simulink model "kurtosis"  (R2012b)
settings: Solver=ode45  StartTime=0.0  StopTime=3171  RelTol=1e-3
libraries: xbsIndex_r4 x3174, casper_library_flow_control x64, casper_library_misc x1, simulink_xsg_bridge x1
(part 7 of 24)

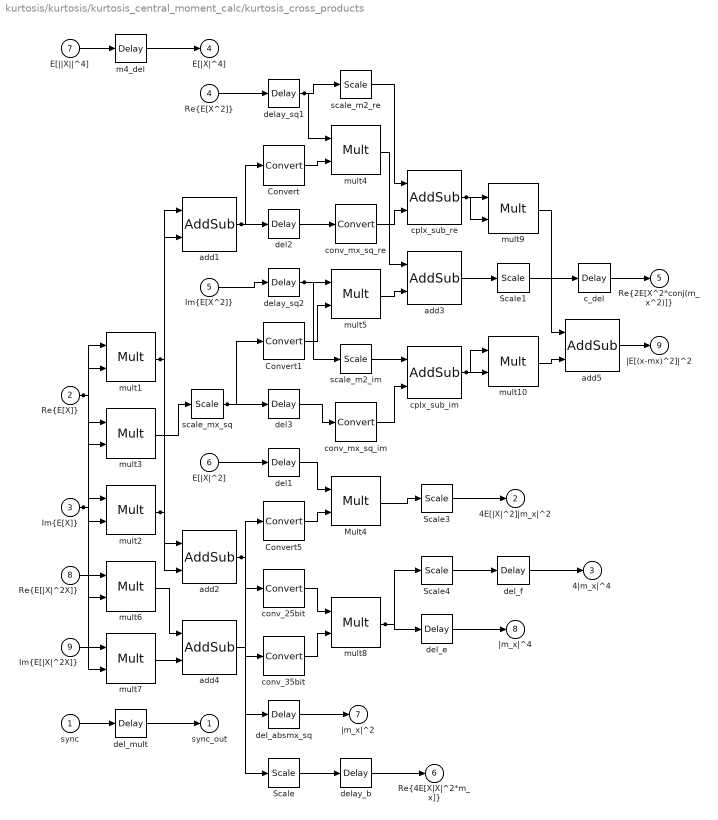
== system kurtosis/kurtosis/kurtosis_central_moment_calc/kurtosis_cross_products ==
  sync : Inport
  "Re{E[X]}" : Inport  Port=2
  "Im{E[X]}" : Inport  Port=3
  "Re{E[X^2]}" : Inport  Port=4
  "Im{E[X^2]}" : Inport  Port=5
  E[|X|^2] : Inport  Port=6
  E[||X||^4] : Inport  Port=7
  "Re{E[|X|^2X]}" : Inport  Port=8
  "Im{E[|X|^2X]}" : Inport  Port=9
  Convert : xbsIndex_r4/Convert  gui_display_data_type=Fixed-point  arith_type="Signed  (2's comp)"  n_bits=25  bin_pt=22  float_type=Single  exp_bits=8  fraction_bits=24  quantization="Round  (unbiased: +/- Inf)"  overflow=Saturate  en=off  latency=1  dbl_ovrd=off  pipeline=off  block_type=convert
  Convert1 : xbsIndex_r4/Convert  gui_display_data_type=Fixed-point  arith_type="Signed  (2's comp)"  n_bits=25  bin_pt=22  float_type=Single  exp_bits=8  fraction_bits=24  quantization="Round  (unbiased: +/- Inf)"  overflow=Saturate  en=off  latency=1  dbl_ovrd=off  pipeline=off  block_type=convert
  Convert5 : xbsIndex_r4/Convert  gui_display_data_type=Fixed-point  arith_type="Signed  (2's comp)"  n_bits=25  bin_pt=22  float_type=Single  exp_bits=8  fraction_bits=24  quantization="Round  (unbiased: +/- Inf)"  overflow=Saturate  en=off  latency=5  dbl_ovrd=off  pipeline=off  block_type=convert
  Mult4 : xbsIndex_r4/Mult  precision=Full  arith_type="Signed  (2's comp)"  n_bits=36  bin_pt=34  quantization=Truncate  overflow=Wrap  en=off  latency=5  dbl_ovrd=off  use_behavioral_HDL=off  opt=Speed  use_embedded=on  optimum_pipeline=off  pipeline=on  use_rpm=on  placement_style=Triangular  block_type=mult
  Scale : xbsIndex_r4/Scale  scale_factor=2  dbl_ovrd=off  block_type=scale
  Scale1 : xbsIndex_r4/Scale  scale_factor=1  dbl_ovrd=off  block_type=scale
  Scale3 : xbsIndex_r4/Scale  scale_factor=2  dbl_ovrd=off  block_type=scale
  Scale4 : xbsIndex_r4/Scale  scale_factor=2  dbl_ovrd=off  block_type=scale
  add1 : xbsIndex_r4/AddSub  mode=Subtraction  use_carryin=off  use_carryout=off  en=off  latency=2  precision=Full  arith_type="Signed  (2's comp)"  n_bits=36  bin_pt=34  quantization=Truncate  overflow=Wrap  dbl_ovrd=off  use_behavioral_HDL=off  hw_selection=Fabric  pipelined=off  block_type=addsub
  add2 : xbsIndex_r4/AddSub  mode=Addition  use_carryin=off  use_carryout=off  en=off  latency=2  precision=Full  arith_type="Signed  (2's comp)"  n_bits=36  bin_pt=34  quantization=Truncate  overflow=Wrap  dbl_ovrd=off  use_behavioral_HDL=off  hw_selection=Fabric  pipelined=off  block_type=addsub
  add3 : xbsIndex_r4/AddSub  mode=Addition  use_carryin=off  use_carryout=off  en=off  latency=2  precision=Full  arith_type="Signed  (2's comp)"  n_bits=36  bin_pt=34  quantization=Truncate  overflow=Wrap  dbl_ovrd=off  use_behavioral_HDL=off  hw_selection=Fabric  pipelined=off  block_type=addsub
  add4 : xbsIndex_r4/AddSub  mode=Addition  use_carryin=off  use_carryout=off  en=off  latency=2  precision=Full  arith_type="Signed  (2's comp)"  n_bits=36  bin_pt=34  quantization=Truncate  overflow=Wrap  dbl_ovrd=off  use_behavioral_HDL=off  hw_selection=Fabric  pipelined=off  block_type=addsub
  add5 : xbsIndex_r4/AddSub  mode=Addition  use_carryin=off  use_carryout=off  en=off  latency=3  precision=Full  arith_type="Signed  (2's comp)"  n_bits=36  bin_pt=34  quantization=Truncate  overflow=Wrap  dbl_ovrd=off  use_behavioral_HDL=off  hw_selection=Fabric  pipelined=off  block_type=addsub
  c_del : xbsIndex_r4/Delay  rst=off  infoeditControl=Selection of Reset will increase slice count due to use of real FFs and instead of SRLs  en=off  latency=4  dbl_ovrd=off  reg_retiming=off  block_type=delay
  conv_25bit : xbsIndex_r4/Convert  gui_display_data_type=Fixed-point  arith_type="Signed  (2's comp)"  n_bits=25  bin_pt=22  float_type=Single  exp_bits=8  fraction_bits=24  quantization="Round  (unbiased: +/- Inf)"  overflow=Saturate  en=off  latency=3  dbl_ovrd=off  pipeline=off  block_type=convert
  conv_35bit : xbsIndex_r4/Convert  gui_display_data_type=Fixed-point  arith_type="Signed  (2's comp)"  n_bits=35  bin_pt=32  float_type=Single  exp_bits=8  fraction_bits=24  quantization="Round  (unbiased: +/- Inf)"  overflow=Saturate  en=off  latency=3  dbl_ovrd=off  pipeline=off  block_type=convert
  conv_mx_sq_im : xbsIndex_r4/Convert  gui_display_data_type=Fixed-point  arith_type="Signed  (2's comp)"  n_bits=35  bin_pt=32  float_type=Single  exp_bits=8  fraction_bits=24  quantization="Round  (unbiased: +/- Inf)"  overflow=Saturate  en=off  latency=0  dbl_ovrd=off  pipeline=off  block_type=convert
  conv_mx_sq_re : xbsIndex_r4/Convert  gui_display_data_type=Fixed-point  arith_type="Signed  (2's comp)"  n_bits=35  bin_pt=32  float_type=Single  exp_bits=8  fraction_bits=24  quantization="Round  (unbiased: +/- Inf)"  overflow=Saturate  en=off  latency=0  dbl_ovrd=off  pipeline=off  block_type=convert
  cplx_sub_im : xbsIndex_r4/AddSub  mode=Subtraction  use_carryin=off  use_carryout=off  en=off  latency=2  precision=Full  arith_type="Signed  (2's comp)"  n_bits=36  bin_pt=34  quantization=Truncate  overflow=Wrap  dbl_ovrd=off  use_behavioral_HDL=off  hw_selection=Fabric  pipelined=off  block_type=addsub
  cplx_sub_re : xbsIndex_r4/AddSub  mode=Subtraction  use_carryin=off  use_carryout=off  en=off  latency=2  precision=Full  arith_type="Signed  (2's comp)"  n_bits=36  bin_pt=34  quantization=Truncate  overflow=Wrap  dbl_ovrd=off  use_behavioral_HDL=off  hw_selection=Fabric  pipelined=off  block_type=addsub
  del1 : xbsIndex_r4/Delay  rst=off  infoeditControl=Selection of Reset will increase slice count due to use of real FFs and instead of SRLs  en=off  latency=10  dbl_ovrd=off  reg_retiming=off  block_type=delay
  del2 : xbsIndex_r4/Delay  rst=off  infoeditControl=Selection of Reset will increase slice count due to use of real FFs and instead of SRLs  en=off  latency=1  dbl_ovrd=off  reg_retiming=off  block_type=delay
  del3 : xbsIndex_r4/Delay  rst=off  infoeditControl=Selection of Reset will increase slice count due to use of real FFs and instead of SRLs  en=off  latency=1  dbl_ovrd=off  reg_retiming=off  block_type=delay
  del_absmx_sq : xbsIndex_r4/Delay  rst=off  infoeditControl=Selection of Reset will increase slice count due to use of real FFs and instead of SRLs  en=off  latency=10  dbl_ovrd=off  reg_retiming=off  block_type=delay
  del_e : xbsIndex_r4/Delay  rst=off  infoeditControl=Selection of Reset will increase slice count due to use of real FFs and instead of SRLs  en=off  latency=2  dbl_ovrd=off  reg_retiming=off  block_type=delay
  del_f : xbsIndex_r4/Delay  rst=off  infoeditControl=Selection of Reset will increase slice count due to use of real FFs and instead of SRLs  en=off  latency=2  dbl_ovrd=off  reg_retiming=off  block_type=delay
  del_mult : xbsIndex_r4/Delay  rst=off  infoeditControl=Selection of Reset will increase slice count due to use of real FFs and instead of SRLs  en=off  latency=15  dbl_ovrd=off  reg_retiming=off  block_type=delay
  delay_b : xbsIndex_r4/Delay  rst=off  infoeditControl=Selection of Reset will increase slice count due to use of real FFs and instead of SRLs  en=off  latency=7  dbl_ovrd=off  reg_retiming=off  block_type=delay
  delay_sq1 : xbsIndex_r4/Delay  rst=off  infoeditControl=Selection of Reset will increase slice count due to use of real FFs and instead of SRLs  en=off  latency=6  dbl_ovrd=off  reg_retiming=off  block_type=delay
  delay_sq2 : xbsIndex_r4/Delay  rst=off  infoeditControl=Selection of Reset will increase slice count due to use of real FFs and instead of SRLs  en=off  latency=6  dbl_ovrd=off  reg_retiming=off  block_type=delay
  m4_del : xbsIndex_r4/Delay  rst=off  infoeditControl=Selection of Reset will increase slice count due to use of real FFs and instead of SRLs  en=off  latency=15  dbl_ovrd=off  reg_retiming=off  block_type=delay
  mult{1..2,4..5} (4 alike) : xbsIndex_r4/Mult  precision=Full  arith_type="Signed  (2's comp)"  n_bits=36  bin_pt=34  quantization=Truncate  overflow=Wrap  en=off  latency=3  dbl_ovrd=off  use_behavioral_HDL=off  opt=Speed  use_embedded=on  optimum_pipeline=off  pipeline=on  use_rpm=on  placement_style=Triangular  block_type=mult
  mult10 : xbsIndex_r4/Mult  precision=Full  arith_type="Signed  (2's comp)"  n_bits=36  bin_pt=34  quantization=Truncate  overflow=Wrap  en=off  latency=4  dbl_ovrd=off  use_behavioral_HDL=off  opt=Speed  use_embedded=on  optimum_pipeline=off  pipeline=on  use_rpm=on  placement_style=Triangular  block_type=mult
  mult3 : xbsIndex_r4/Mult  precision=Full  arith_type="Signed  (2's comp)"  n_bits=36  bin_pt=34  quantization=Truncate  overflow=Wrap  en=off  latency=5  dbl_ovrd=off  use_behavioral_HDL=off  opt=Speed  use_embedded=on  optimum_pipeline=off  pipeline=on  use_rpm=on  placement_style=Triangular  block_type=mult
  mult6 : xbsIndex_r4/Mult  precision=Full  arith_type="Signed  (2's comp)"  n_bits=36  bin_pt=34  quantization=Truncate  overflow=Wrap  en=off  latency=6  dbl_ovrd=off  use_behavioral_HDL=off  opt=Speed  use_embedded=on  optimum_pipeline=off  pipeline=on  use_rpm=on  placement_style=Triangular  block_type=mult
  mult7 : xbsIndex_r4/Mult  precision=Full  arith_type="Signed  (2's comp)"  n_bits=36  bin_pt=34  quantization=Truncate  overflow=Wrap  en=off  latency=6  dbl_ovrd=off  use_behavioral_HDL=off  opt=Speed  use_embedded=on  optimum_pipeline=off  pipeline=on  use_rpm=on  placement_style=Triangular  block_type=mult
  mult8 : xbsIndex_r4/Mult  precision=Full  arith_type="Signed  (2's comp)"  n_bits=36  bin_pt=34  quantization=Truncate  overflow=Wrap  en=off  latency=5  dbl_ovrd=off  use_behavioral_HDL=off  opt=Speed  use_embedded=on  optimum_pipeline=off  pipeline=on  use_rpm=on  placement_style=Triangular  block_type=mult
  mult9 : xbsIndex_r4/Mult  precision=Full  arith_type="Signed  (2's comp)"  n_bits=36  bin_pt=34  quantization=Truncate  overflow=Wrap  en=off  latency=4  dbl_ovrd=off  use_behavioral_HDL=off  opt=Speed  use_embedded=on  optimum_pipeline=off  pipeline=on  use_rpm=on  placement_style=Triangular  block_type=mult
  scale_m2_im : xbsIndex_r4/Scale  scale_factor=-10  dbl_ovrd=off  block_type=scale
  scale_m2_re : xbsIndex_r4/Scale  scale_factor=-10  dbl_ovrd=off  block_type=scale
  scale_mx_sq : xbsIndex_r4/Scale  scale_factor=1  dbl_ovrd=off  block_type=scale
  sync_out : Outport
  4E[|X|^2]|m_x|^2 : Outport  Port=2
  4|m_x|^4 : Outport  Port=3
  E[|X|^4] : Outport  Port=4
  "Re{2E[X^2*conj(m_x^2)]}" : Outport  Port=5
  "Re{4E[X|X|^2*m_x]}" : Outport  Port=6
  |m_x|^2 : Outport  Port=7
  |m_x|^4 : Outport  Port=8
  |E[(x-mx)^2]|^2 : Outport  Port=9
  wires:
  "Re{E[X]}"/1 -> mult6/2, mult3/1, mult1/2, mult1/1
  "Im{E[X]}"/1 -> mult7/2, mult3/2, mult2/2, mult2/1
  mult1/1 -> add2/1, add1/1
  mult2/1 -> add2/2, add1/2
  add1/1 -> del2/1, Convert/1
  scale_mx_sq/1 -> del3/1, Convert1/1
  delay_sq1/1 -> scale_m2_re/1, mult4/1
  delay_sq2/1 -> scale_m2_im/1, mult5/1
  add2/1 -> del_absmx_sq/1, Convert5/1, conv_35bit/1, conv_25bit/1
  mult8/1 -> Scale4/1, del_e/1
  cplx_sub_re/1 -> mult9/2, mult9/1
  cplx_sub_im/1 -> mult10/2, mult10/1
  del_absmx_sq/1 -> |m_x|^2/1
  add5/1 -> |E[(x-mx)^2]|^2/1
  del_f/1 -> 4|m_x|^4/1
  del_e/1 -> |m_x|^4/1
  Scale3/1 -> 4E[|X|^2]|m_x|^2/1
  c_del/1 -> "Re{2E[X^2*conj(m_x^2)]}"/1
  delay_b/1 -> "Re{4E[X|X|^2*m_x]}"/1
  m4_del/1 -> E[|X|^4]/1
  E[||X||^4]/1 -> m4_del/1
  del_mult/1 -> sync_out/1
  sync/1 -> del_mult/1
  mult10/1 -> add5/2
  mult9/1 -> add5/1
  conv_mx_sq_im/1 -> cplx_sub_im/2
  scale_m2_im/1 -> cplx_sub_im/1
  conv_mx_sq_re/1 -> cplx_sub_re/2
  scale_m2_re/1 -> cplx_sub_re/1
  del3/1 -> conv_mx_sq_im/1
  del2/1 -> conv_mx_sq_re/1
  Scale4/1 -> del_f/1
  Mult4/1 -> Scale3/1
  Convert5/1 -> Mult4/2
  del1/1 -> Mult4/1
  E[|X|^2]/1 -> del1/1
  Scale1/1 -> c_del/1
  add3/1 -> Scale1/1
  Scale/1 -> delay_b/1
  add4/1 -> Scale/1
  conv_35bit/1 -> mult8/2
  conv_25bit/1 -> mult8/1
  mult7/1 -> add4/2
  mult6/1 -> add4/1
  "Im{E[|X|^2X]}"/1 -> mult7/1
  "Re{E[|X|^2X]}"/1 -> mult6/1
  mult5/1 -> add3/2
  mult4/1 -> add3/1
  Convert1/1 -> mult5/2
  Convert/1 -> mult4/2
  "Im{E[X^2]}"/1 -> delay_sq2/1
  "Re{E[X^2]}"/1 -> delay_sq1/1
  mult3/1 -> scale_mx_sq/1

== system kurtosis/kurtosis/kurtosis_central_moment_calc/kurtosis_den ==
  E[|X|^2] : Inport
  |m_x|^2 : Inport  Port=2
  Sub : xbsIndex_r4/AddSub  mode=Subtraction  use_carryin=off  use_carryout=off  en=off  latency=4  precision=Full  arith_type="Signed  (2's comp)"  n_bits=36  bin_pt=34  quantization=Truncate  overflow=Wrap  dbl_ovrd=off  use_behavioral_HDL=off  hw_selection=Fabric  pipelined=off  block_type=addsub
  conv : xbsIndex_r4/Convert  gui_display_data_type=Fixed-point  arith_type="Signed  (2's comp)"  n_bits=64  bin_pt=56  float_type=Single  exp_bits=8  fraction_bits=24  quantization="Round  (unbiased: +/- Inf)"  overflow=Saturate  en=off  latency=1  dbl_ovrd=off  pipeline=off  block_type=convert
  scale : xbsIndex_r4/Scale  scale_factor=-10  dbl_ovrd=off  block_type=scale
  square : xbsIndex_r4/Mult  precision=Full  arith_type="Signed  (2's comp)"  n_bits=36  bin_pt=34  quantization=Truncate  overflow=Wrap  en=off  latency=5  dbl_ovrd=off  use_behavioral_HDL=off  opt=Speed  use_embedded=on  optimum_pipeline=off  pipeline=on  use_rpm=on  placement_style=Triangular  block_type=mult
  square_conv_25bit : xbsIndex_r4/Convert  gui_display_data_type=Fixed-point  arith_type="Signed  (2's comp)"  n_bits=25  bin_pt=21  float_type=Single  exp_bits=8  fraction_bits=24  quantization="Round  (unbiased: +/- Inf)"  overflow=Saturate  en=off  latency=3  dbl_ovrd=off  pipeline=off  block_type=convert
  square_conv_35bit : xbsIndex_r4/Convert  gui_display_data_type=Fixed-point  arith_type="Signed  (2's comp)"  n_bits=35  bin_pt=31  float_type=Single  exp_bits=8  fraction_bits=24  quantization="Round  (unbiased: +/- Inf)"  overflow=Saturate  en=off  latency=3  dbl_ovrd=off  pipeline=off  block_type=convert
  E[|X-m_x|^2]^2 : Outport
  wires:
  Sub/1 -> square_conv_25bit/1, square_conv_35bit/1
  conv/1 -> E[|X-m_x|^2]^2/1
  square/1 -> conv/1
  square_conv_25bit/1 -> square/2
  square_conv_35bit/1 -> square/1
  |m_x|^2/1 -> Sub/2
  scale/1 -> Sub/1
  E[|X|^2]/1 -> scale/1

== system kurtosis/kurtosis/kurtosis_central_moment_calc/kurtosis_num ==
  sync : Inport
  4E[|X|^2]|m_x|^2 : Inport  Port=2
  4|m_x|^4 : Inport  Port=3
  E[|X|^4] : Inport  Port=4
  "Re{2E[X^2*conj(m_x^2)]}" : Inport  Port=5
  "Re{4E[X|X|^2*m_x]}" : Inport  Port=6
  |m_x|^4 : Inport  Port=7
  |E[(x-mx)^2]|^2 : Inport  Port=8
  a_del : xbsIndex_r4/Delay  rst=off  infoeditControl=Selection of Reset will increase slice count due to use of real FFs and instead of SRLs  en=off  latency=4  dbl_ovrd=off  reg_retiming=off  block_type=delay
  add : xbsIndex_r4/AddSub  mode=Addition  use_carryin=off  use_carryout=off  en=off  latency=4  precision=Full  arith_type="Signed  (2's comp)"  n_bits=36  bin_pt=34  quantization=Truncate  overflow=Wrap  dbl_ovrd=off  use_behavioral_HDL=off  hw_selection=Fabric  pipelined=off  block_type=addsub
  add_aef : xbsIndex_r4/AddSub  mode=Addition  use_carryin=off  use_carryout=off  en=off  latency=4  precision=Full  arith_type="Signed  (2's comp)"  n_bits=36  bin_pt=34  quantization=Truncate  overflow=Wrap  dbl_ovrd=off  use_behavioral_HDL=off  hw_selection=Fabric  pipelined=off  block_type=addsub
  add_dcb : xbsIndex_r4/AddSub  mode=Addition  use_carryin=off  use_carryout=off  en=off  latency=4  precision=Full  arith_type="Signed  (2's comp)"  n_bits=36  bin_pt=34  quantization=Truncate  overflow=Wrap  dbl_ovrd=off  use_behavioral_HDL=off  hw_selection=Fabric  pipelined=off  block_type=addsub
  conv : xbsIndex_r4/Convert  gui_display_data_type=Fixed-point  arith_type="Signed  (2's comp)"  n_bits=96  bin_pt=84  float_type=Single  exp_bits=8  fraction_bits=24  quantization="Round  (unbiased: +/- Inf)"  overflow=Saturate  en=off  latency=1  dbl_ovrd=off  pipeline=off  block_type=convert
  scale_a : xbsIndex_r4/Scale  scale_factor=-10  dbl_ovrd=off  block_type=scale
  scale_b : xbsIndex_r4/Scale  scale_factor=-10  dbl_ovrd=off  block_type=scale
  scale_c : xbsIndex_r4/Scale  scale_factor=-10  dbl_ovrd=off  block_type=scale
  scale_d : xbsIndex_r4/Scale  scale_factor=-10  dbl_ovrd=off  block_type=scale
  sub_cb : xbsIndex_r4/AddSub  mode=Subtraction  use_carryin=off  use_carryout=off  en=off  latency=4  precision=Full  arith_type="Signed  (2's comp)"  n_bits=36  bin_pt=34  quantization=Truncate  overflow=Wrap  dbl_ovrd=off  use_behavioral_HDL=off  hw_selection=Fabric  pipelined=off  block_type=addsub
  sub_dh : xbsIndex_r4/AddSub  mode=Subtraction  use_carryin=off  use_carryout=off  en=off  latency=4  precision=Full  arith_type="Signed  (2's comp)"  n_bits=36  bin_pt=34  quantization=Truncate  overflow=Wrap  dbl_ovrd=off  use_behavioral_HDL=off  hw_selection=Fabric  pipelined=off  block_type=addsub
  sub_ef : xbsIndex_r4/AddSub  mode=Subtraction  use_carryin=off  use_carryout=off  en=off  latency=4  precision=Full  arith_type="Signed  (2's comp)"  n_bits=36  bin_pt=34  quantization=Truncate  overflow=Wrap  dbl_ovrd=off  use_behavioral_HDL=off  hw_selection=Fabric  pipelined=off  block_type=addsub
  sync_del : xbsIndex_r4/Delay  rst=off  infoeditControl=Selection of Reset will increase slice count due to use of real FFs and instead of SRLs  en=off  latency=13  dbl_ovrd=off  reg_retiming=off  block_type=delay
  sync_out : Outport
  E[|X-m_x|^4] : Outport  Port=2
  wires:
  sync_del/1 -> sync_out/1
  conv/1 -> E[|X-m_x|^4]/1
  add/1 -> conv/1
  add_dcb/1 -> add/2
  add_aef/1 -> add/1
  sub_cb/1 -> add_dcb/2
  sub_dh/1 -> add_dcb/1
  a_del/1 -> add_aef/2
  sub_ef/1 -> add_aef/1
  scale_a/1 -> a_del/1
  |E[(x-mx)^2]|^2/1 -> sub_dh/2
  scale_d/1 -> sub_dh/1
  scale_b/1 -> sub_cb/2
  scale_c/1 -> sub_cb/1
  4|m_x|^4/1 -> sub_ef/2
  |m_x|^4/1 -> sub_ef/1
  4E[|X|^2]|m_x|^2/1 -> scale_d/1
  "Re{2E[X^2*conj(m_x^2)]}"/1 -> scale_c/1
  "Re{4E[X|X|^2*m_x]}"/1 -> scale_b/1
  E[|X|^4]/1 -> scale_a/1
  sync/1 -> sync_del/1

== system kurtosis/kurtosis/kurtosis_origin_moments_1/abs_x_sq ==
  c : Inport
  c_to_ri : Subsystem
  imag_square : xbsIndex_r4/Mult  precision=Full  arith_type="Signed  (2's comp)"  n_bits=16  bin_pt=14  quantization=Truncate  overflow=Wrap  en=off  latency=3  dbl_ovrd=off  use_behavioral_HDL=off  opt=Speed  use_embedded=on  optimum_pipeline=off  pipeline=on  use_rpm=on  placement_style=Rectangular shape  block_type=mult
  power_adder : xbsIndex_r4/AddSub  mode=Addition  use_carryin=off  use_carryout=off  en=off  latency=2  precision=Full  arith_type=Unsigned  n_bits=16  bin_pt=14  quantization=Truncate  overflow=Wrap  dbl_ovrd=off  use_behavioral_HDL=on  hw_selection=Fabric  pipelined=off  use_rpm=on  block_type=addsub
  real_square : xbsIndex_r4/Mult  precision=Full  arith_type="Signed  (2's comp)"  n_bits=16  bin_pt=14  quantization=Truncate  overflow=Wrap  en=off  latency=3  dbl_ovrd=off  use_behavioral_HDL=off  opt=Speed  use_embedded=on  optimum_pipeline=off  pipeline=on  use_rpm=on  placement_style=Triangular  block_type=mult
  power : Outport
  wires:
  c_to_ri/2(im) -> imag_square/2, imag_square/1
  c_to_ri/1(re) -> real_square/2, real_square/1
  real_square/1 -> power_adder/1
  power_adder/1 -> power/1
  imag_square/1 -> power_adder/2
  c/1 -> c_to_ri/1(c)

== system kurtosis/kurtosis/kurtosis_origin_moments_1/c_to_ri_xin ==
  c : Inport
  force_im : xbsIndex_r4/Reinterpret  force_arith_type=on  arith_type="Signed  (2's comp)"  force_bin_pt=on  bin_pt=17  block_type=reinterpret
  force_re : xbsIndex_r4/Reinterpret  force_arith_type=on  arith_type="Signed  (2's comp)"  force_bin_pt=on  bin_pt=17  block_type=reinterpret
  slice_im : xbsIndex_r4/Slice  nbits=18  boolean_output=off  mode=Lower Bit Location + Width  bit1=0  base1=MSB of Input  bit0=0  base0=LSB of Input  dbl_ovrd=off  block_type=slice
  slice_re : xbsIndex_r4/Slice  nbits=18  boolean_output=off  mode=Upper Bit Location + Width  bit1=0  base1=MSB of Input  bit0=0  base0=LSB of Input  dbl_ovrd=off  block_type=slice
  re : Outport
  im : Outport  Port=2
  wires:
  c/1 -> slice_im/1, slice_re/1
  force_im/1 -> im/1
  slice_im/1 -> force_im/1
  force_re/1 -> re/1
  slice_re/1 -> force_re/1

== system kurtosis/kurtosis/kurtosis_origin_moments_1/cplx_sq ==
  a : Inport
  b : Inport  Port=2
  AddSub : xbsIndex_r4/AddSub  mode=Subtraction  use_carryin=off  use_carryout=off  en=off  latency=2  precision=Full  arith_type=Unsigned  n_bits=16  bin_pt=14  quantization=Truncate  overflow=Wrap  dbl_ovrd=off  use_behavioral_HDL=on  hw_selection=Fabric  pipelined=off  block_type=addsub
  AddSub1 : xbsIndex_r4/AddSub  mode=Addition  use_carryin=off  use_carryout=off  en=off  latency=2  precision=Full  arith_type=Unsigned  n_bits=16  bin_pt=14  quantization=Truncate  overflow=Wrap  dbl_ovrd=off  use_behavioral_HDL=on  hw_selection=Fabric  pipelined=off  block_type=addsub
  a_input_c_to_ri : Subsystem
  b_input_c_to_ri : Subsystem
  c_output_ri_to_c : Subsystem
  convert0 : xbsIndex_r4/Convert  gui_display_data_type=Fixed-point  arith_type="Signed  (2's comp)"  n_bits=37  bin_pt=34  float_type=Single  exp_bits=8  fraction_bits=24  quantization=Truncate  overflow=Wrap  en=off  latency=1  dbl_ovrd=off  pipeline=on  block_type=convert
  convert1 : xbsIndex_r4/Convert  gui_display_data_type=Fixed-point  arith_type="Signed  (2's comp)"  n_bits=37  bin_pt=34  float_type=Single  exp_bits=8  fraction_bits=24  quantization=Truncate  overflow=Wrap  en=off  latency=1  dbl_ovrd=off  pipeline=on  block_type=convert
  mults : Subsystem
  c : Outport
  wires:
  a_input_c_to_ri/1(re) -> mults/7(a4), mults/1(a1)  "a_re"
  b_input_c_to_ri/1(re) -> mults/6(b3), mults/2(b1)  "b_re"
  a_input_c_to_ri/2(im) -> mults/5(a3), mults/3(a2)  "a_im"
  b_input_c_to_ri/2(im) -> mults/8(b4), mults/4(b2)  "b_im"
  convert1/1 -> c_output_ri_to_c/2(im)  "c_im"
  AddSub1/1 -> convert1/1
  convert0/1 -> c_output_ri_to_c/1(re)  "c_re"
  AddSub/1 -> convert0/1
  mults/4(c4) -> AddSub1/2
  mults/3(c3) -> AddSub1/1
  mults/2(c2) -> AddSub/2
  mults/1(c1) -> AddSub/1
  c_output_ri_to_c/1(c) -> c/1
  b/1 -> b_input_c_to_ri/1(c)
  a/1 -> a_input_c_to_ri/1(c)

== system kurtosis/kurtosis/kurtosis_origin_moments_1/ri_to_c_x_3rd ==
  re : Inport
  im : Inport  Port=2
  concat : xbsIndex_r4/Concat  num_inputs=2  dbl_ovrd=off  block_type=concat
  force_im : xbsIndex_r4/Reinterpret  force_arith_type=on  arith_type=Unsigned  force_bin_pt=on  bin_pt=0  block_type=reinterpret
  force_re : xbsIndex_r4/Reinterpret  force_arith_type=on  arith_type=Unsigned  force_bin_pt=on  bin_pt=0  block_type=reinterpret
  c : Outport
  wires:
  force_re/1 -> concat/1
  re/1 -> force_re/1
  force_im/1 -> concat/2
  im/1 -> force_im/1
  concat/1 -> c/1

== system kurtosis/kurtosis/kurtosis_origin_moments_2/abs_x_sq ==
  c : Inport
  c_to_ri : Subsystem
  imag_square : xbsIndex_r4/Mult  precision=Full  arith_type="Signed  (2's comp)"  n_bits=16  bin_pt=14  quantization=Truncate  overflow=Wrap  en=off  latency=3  dbl_ovrd=off  use_behavioral_HDL=off  opt=Speed  use_embedded=on  optimum_pipeline=off  pipeline=on  use_rpm=on  placement_style=Rectangular shape  block_type=mult
  power_adder : xbsIndex_r4/AddSub  mode=Addition  use_carryin=off  use_carryout=off  en=off  latency=2  precision=Full  arith_type=Unsigned  n_bits=16  bin_pt=14  quantization=Truncate  overflow=Wrap  dbl_ovrd=off  use_behavioral_HDL=on  hw_selection=Fabric  pipelined=off  use_rpm=on  block_type=addsub
  real_square : xbsIndex_r4/Mult  precision=Full  arith_type="Signed  (2's comp)"  n_bits=16  bin_pt=14  quantization=Truncate  overflow=Wrap  en=off  latency=3  dbl_ovrd=off  use_behavioral_HDL=off  opt=Speed  use_embedded=on  optimum_pipeline=off  pipeline=on  use_rpm=on  placement_style=Triangular  block_type=mult
  power : Outport
  wires:
  c_to_ri/2(im) -> imag_square/2, imag_square/1
  c_to_ri/1(re) -> real_square/2, real_square/1
  real_square/1 -> power_adder/1
  power_adder/1 -> power/1
  imag_square/1 -> power_adder/2
  c/1 -> c_to_ri/1(c)

== system kurtosis/kurtosis/kurtosis_origin_moments_2/c_to_ri_xin ==
  c : Inport
  force_im : xbsIndex_r4/Reinterpret  force_arith_type=on  arith_type="Signed  (2's comp)"  force_bin_pt=on  bin_pt=17  block_type=reinterpret
  force_re : xbsIndex_r4/Reinterpret  force_arith_type=on  arith_type="Signed  (2's comp)"  force_bin_pt=on  bin_pt=17  block_type=reinterpret
  slice_im : xbsIndex_r4/Slice  nbits=18  boolean_output=off  mode=Lower Bit Location + Width  bit1=0  base1=MSB of Input  bit0=0  base0=LSB of Input  dbl_ovrd=off  block_type=slice
  slice_re : xbsIndex_r4/Slice  nbits=18  boolean_output=off  mode=Upper Bit Location + Width  bit1=0  base1=MSB of Input  bit0=0  base0=LSB of Input  dbl_ovrd=off  block_type=slice
  re : Outport
  im : Outport  Port=2
  wires:
  c/1 -> slice_im/1, slice_re/1
  force_im/1 -> im/1
  slice_im/1 -> force_im/1
  force_re/1 -> re/1
  slice_re/1 -> force_re/1

== system kurtosis/kurtosis/kurtosis_origin_moments_2/cplx_sq ==
  a : Inport
  b : Inport  Port=2
  AddSub : xbsIndex_r4/AddSub  mode=Subtraction  use_carryin=off  use_carryout=off  en=off  latency=2  precision=Full  arith_type=Unsigned  n_bits=16  bin_pt=14  quantization=Truncate  overflow=Wrap  dbl_ovrd=off  use_behavioral_HDL=on  hw_selection=Fabric  pipelined=off  block_type=addsub
  AddSub1 : xbsIndex_r4/AddSub  mode=Addition  use_carryin=off  use_carryout=off  en=off  latency=2  precision=Full  arith_type=Unsigned  n_bits=16  bin_pt=14  quantization=Truncate  overflow=Wrap  dbl_ovrd=off  use_behavioral_HDL=on  hw_selection=Fabric  pipelined=off  block_type=addsub
  a_input_c_to_ri : Subsystem
  b_input_c_to_ri : Subsystem
  c_output_ri_to_c : Subsystem
  convert0 : xbsIndex_r4/Convert  gui_display_data_type=Fixed-point  arith_type="Signed  (2's comp)"  n_bits=37  bin_pt=34  float_type=Single  exp_bits=8  fraction_bits=24  quantization=Truncate  overflow=Wrap  en=off  latency=1  dbl_ovrd=off  pipeline=on  block_type=convert
  convert1 : xbsIndex_r4/Convert  gui_display_data_type=Fixed-point  arith_type="Signed  (2's comp)"  n_bits=37  bin_pt=34  float_type=Single  exp_bits=8  fraction_bits=24  quantization=Truncate  overflow=Wrap  en=off  latency=1  dbl_ovrd=off  pipeline=on  block_type=convert
  mults : Subsystem
  c : Outport
  wires:
  a_input_c_to_ri/1(re) -> mults/7(a4), mults/1(a1)  "a_re"
  b_input_c_to_ri/1(re) -> mults/6(b3), mults/2(b1)  "b_re"
  a_input_c_to_ri/2(im) -> mults/5(a3), mults/3(a2)  "a_im"
  b_input_c_to_ri/2(im) -> mults/8(b4), mults/4(b2)  "b_im"
  convert1/1 -> c_output_ri_to_c/2(im)  "c_im"
  AddSub1/1 -> convert1/1
  convert0/1 -> c_output_ri_to_c/1(re)  "c_re"
  AddSub/1 -> convert0/1
  mults/4(c4) -> AddSub1/2
  mults/3(c3) -> AddSub1/1
  mults/2(c2) -> AddSub/2
  mults/1(c1) -> AddSub/1
  c_output_ri_to_c/1(c) -> c/1
  b/1 -> b_input_c_to_ri/1(c)
  a/1 -> a_input_c_to_ri/1(c)

== system kurtosis/kurtosis/kurtosis_origin_moments_2/ri_to_c_x_3rd ==
  re : Inport
  im : Inport  Port=2
  concat : xbsIndex_r4/Concat  num_inputs=2  dbl_ovrd=off  block_type=concat
  force_im : xbsIndex_r4/Reinterpret  force_arith_type=on  arith_type=Unsigned  force_bin_pt=on  bin_pt=0  block_type=reinterpret
  force_re : xbsIndex_r4/Reinterpret  force_arith_type=on  arith_type=Unsigned  force_bin_pt=on  bin_pt=0  block_type=reinterpret
  c : Outport
  wires:
  force_re/1 -> concat/1
  re/1 -> force_re/1
  force_im/1 -> concat/2
  im/1 -> force_im/1
  concat/1 -> c/1

== system kurtosis/kurtosis/kurtosis_origin_moments_3/abs_x_sq ==
  c : Inport
  c_to_ri : Subsystem
  imag_square : xbsIndex_r4/Mult  precision=Full  arith_type="Signed  (2's comp)"  n_bits=16  bin_pt=14  quantization=Truncate  overflow=Wrap  en=off  latency=3  dbl_ovrd=off  use_behavioral_HDL=off  opt=Speed  use_embedded=on  optimum_pipeline=off  pipeline=on  use_rpm=on  placement_style=Rectangular shape  block_type=mult
  power_adder : xbsIndex_r4/AddSub  mode=Addition  use_carryin=off  use_carryout=off  en=off  latency=2  precision=Full  arith_type=Unsigned  n_bits=16  bin_pt=14  quantization=Truncate  overflow=Wrap  dbl_ovrd=off  use_behavioral_HDL=on  hw_selection=Fabric  pipelined=off  use_rpm=on  block_type=addsub
  real_square : xbsIndex_r4/Mult  precision=Full  arith_type="Signed  (2's comp)"  n_bits=16  bin_pt=14  quantization=Truncate  overflow=Wrap  en=off  latency=3  dbl_ovrd=off  use_behavioral_HDL=off  opt=Speed  use_embedded=on  optimum_pipeline=off  pipeline=on  use_rpm=on  placement_style=Triangular  block_type=mult
  power : Outport
  wires:
  c_to_ri/2(im) -> imag_square/2, imag_square/1
  c_to_ri/1(re) -> real_square/2, real_square/1
  real_square/1 -> power_adder/1
  power_adder/1 -> power/1
  imag_square/1 -> power_adder/2
  c/1 -> c_to_ri/1(c)

== system kurtosis/kurtosis/kurtosis_origin_moments_3/c_to_ri_xin ==
  c : Inport
  force_im : xbsIndex_r4/Reinterpret  force_arith_type=on  arith_type="Signed  (2's comp)"  force_bin_pt=on  bin_pt=17  block_type=reinterpret
  force_re : xbsIndex_r4/Reinterpret  force_arith_type=on  arith_type="Signed  (2's comp)"  force_bin_pt=on  bin_pt=17  block_type=reinterpret
  slice_im : xbsIndex_r4/Slice  nbits=18  boolean_output=off  mode=Lower Bit Location + Width  bit1=0  base1=MSB of Input  bit0=0  base0=LSB of Input  dbl_ovrd=off  block_type=slice
  slice_re : xbsIndex_r4/Slice  nbits=18  boolean_output=off  mode=Upper Bit Location + Width  bit1=0  base1=MSB of Input  bit0=0  base0=LSB of Input  dbl_ovrd=off  block_type=slice
  re : Outport
  im : Outport  Port=2
  wires:
  c/1 -> slice_im/1, slice_re/1
  force_im/1 -> im/1
  slice_im/1 -> force_im/1
  force_re/1 -> re/1
  slice_re/1 -> force_re/1

== system kurtosis/kurtosis/kurtosis_origin_moments_3/cplx_sq ==
  a : Inport
  b : Inport  Port=2
  AddSub : xbsIndex_r4/AddSub  mode=Subtraction  use_carryin=off  use_carryout=off  en=off  latency=2  precision=Full  arith_type=Unsigned  n_bits=16  bin_pt=14  quantization=Truncate  overflow=Wrap  dbl_ovrd=off  use_behavioral_HDL=on  hw_selection=Fabric  pipelined=off  block_type=addsub
  AddSub1 : xbsIndex_r4/AddSub  mode=Addition  use_carryin=off  use_carryout=off  en=off  latency=2  precision=Full  arith_type=Unsigned  n_bits=16  bin_pt=14  quantization=Truncate  overflow=Wrap  dbl_ovrd=off  use_behavioral_HDL=on  hw_selection=Fabric  pipelined=off  block_type=addsub
  a_input_c_to_ri : Subsystem
  b_input_c_to_ri : Subsystem
  c_output_ri_to_c : Subsystem
  convert0 : xbsIndex_r4/Convert  gui_display_data_type=Fixed-point  arith_type="Signed  (2's comp)"  n_bits=37  bin_pt=34  float_type=Single  exp_bits=8  fraction_bits=24  quantization=Truncate  overflow=Wrap  en=off  latency=1  dbl_ovrd=off  pipeline=on  block_type=convert
  convert1 : xbsIndex_r4/Convert  gui_display_data_type=Fixed-point  arith_type="Signed  (2's comp)"  n_bits=37  bin_pt=34  float_type=Single  exp_bits=8  fraction_bits=24  quantization=Truncate  overflow=Wrap  en=off  latency=1  dbl_ovrd=off  pipeline=on  block_type=convert
  mults : Subsystem
  c : Outport
  wires:
  a_input_c_to_ri/1(re) -> mults/7(a4), mults/1(a1)  "a_re"
  b_input_c_to_ri/1(re) -> mults/6(b3), mults/2(b1)  "b_re"
  a_input_c_to_ri/2(im) -> mults/5(a3), mults/3(a2)  "a_im"
  b_input_c_to_ri/2(im) -> mults/8(b4), mults/4(b2)  "b_im"
  convert1/1 -> c_output_ri_to_c/2(im)  "c_im"
  AddSub1/1 -> convert1/1
  convert0/1 -> c_output_ri_to_c/1(re)  "c_re"
  AddSub/1 -> convert0/1
  mults/4(c4) -> AddSub1/2
  mults/3(c3) -> AddSub1/1
  mults/2(c2) -> AddSub/2
  mults/1(c1) -> AddSub/1
  c_output_ri_to_c/1(c) -> c/1
  b/1 -> b_input_c_to_ri/1(c)
  a/1 -> a_input_c_to_ri/1(c)

== system kurtosis/kurtosis/kurtosis_origin_moments_3/ri_to_c_x_3rd ==
  re : Inport
  im : Inport  Port=2
  concat : xbsIndex_r4/Concat  num_inputs=2  dbl_ovrd=off  block_type=concat
  force_im : xbsIndex_r4/Reinterpret  force_arith_type=on  arith_type=Unsigned  force_bin_pt=on  bin_pt=0  block_type=reinterpret
  force_re : xbsIndex_r4/Reinterpret  force_arith_type=on  arith_type=Unsigned  force_bin_pt=on  bin_pt=0  block_type=reinterpret
  c : Outport
  wires:
  force_re/1 -> concat/1
  re/1 -> force_re/1
  force_im/1 -> concat/2
  im/1 -> force_im/1
  concat/1 -> c/1

== system kurtosis/kurtosis/kurtosis_origin_moments_4/abs_x_sq ==
  c : Inport
  c_to_ri : Subsystem
  imag_square : xbsIndex_r4/Mult  precision=Full  arith_type="Signed  (2's comp)"  n_bits=16  bin_pt=14  quantization=Truncate  overflow=Wrap  en=off  latency=3  dbl_ovrd=off  use_behavioral_HDL=off  opt=Speed  use_embedded=on  optimum_pipeline=off  pipeline=on  use_rpm=on  placement_style=Rectangular shape  block_type=mult
  power_adder : xbsIndex_r4/AddSub  mode=Addition  use_carryin=off  use_carryout=off  en=off  latency=2  precision=Full  arith_type=Unsigned  n_bits=16  bin_pt=14  quantization=Truncate  overflow=Wrap  dbl_ovrd=off  use_behavioral_HDL=on  hw_selection=Fabric  pipelined=off  use_rpm=on  block_type=addsub
  real_square : xbsIndex_r4/Mult  precision=Full  arith_type="Signed  (2's comp)"  n_bits=16  bin_pt=14  quantization=Truncate  overflow=Wrap  en=off  latency=3  dbl_ovrd=off  use_behavioral_HDL=off  opt=Speed  use_embedded=on  optimum_pipeline=off  pipeline=on  use_rpm=on  placement_style=Triangular  block_type=mult
  power : Outport
  wires:
  c_to_ri/2(im) -> imag_square/2, imag_square/1
  c_to_ri/1(re) -> real_square/2, real_square/1
  real_square/1 -> power_adder/1
  power_adder/1 -> power/1
  imag_square/1 -> power_adder/2
  c/1 -> c_to_ri/1(c)

== system kurtosis/kurtosis/kurtosis_origin_moments_4/c_to_ri_xin ==
  c : Inport
  force_im : xbsIndex_r4/Reinterpret  force_arith_type=on  arith_type="Signed  (2's comp)"  force_bin_pt=on  bin_pt=17  block_type=reinterpret
  force_re : xbsIndex_r4/Reinterpret  force_arith_type=on  arith_type="Signed  (2's comp)"  force_bin_pt=on  bin_pt=17  block_type=reinterpret
  slice_im : xbsIndex_r4/Slice  nbits=18  boolean_output=off  mode=Lower Bit Location + Width  bit1=0  base1=MSB of Input  bit0=0  base0=LSB of Input  dbl_ovrd=off  block_type=slice
  slice_re : xbsIndex_r4/Slice  nbits=18  boolean_output=off  mode=Upper Bit Location + Width  bit1=0  base1=MSB of Input  bit0=0  base0=LSB of Input  dbl_ovrd=off  block_type=slice
  re : Outport
  im : Outport  Port=2
  wires:
  c/1 -> slice_im/1, slice_re/1
  force_im/1 -> im/1
  slice_im/1 -> force_im/1
  force_re/1 -> re/1
  slice_re/1 -> force_re/1

== system kurtosis/kurtosis/kurtosis_origin_moments_4/cplx_sq ==
  a : Inport
  b : Inport  Port=2
  AddSub : xbsIndex_r4/AddSub  mode=Subtraction  use_carryin=off  use_carryout=off  en=off  latency=2  precision=Full  arith_type=Unsigned  n_bits=16  bin_pt=14  quantization=Truncate  overflow=Wrap  dbl_ovrd=off  use_behavioral_HDL=on  hw_selection=Fabric  pipelined=off  block_type=addsub
  AddSub1 : xbsIndex_r4/AddSub  mode=Addition  use_carryin=off  use_carryout=off  en=off  latency=2  precision=Full  arith_type=Unsigned  n_bits=16  bin_pt=14  quantization=Truncate  overflow=Wrap  dbl_ovrd=off  use_behavioral_HDL=on  hw_selection=Fabric  pipelined=off  block_type=addsub
  a_input_c_to_ri : Subsystem
  b_input_c_to_ri : Subsystem
  c_output_ri_to_c : Subsystem
  convert0 : xbsIndex_r4/Convert  gui_display_data_type=Fixed-point  arith_type="Signed  (2's comp)"  n_bits=37  bin_pt=34  float_type=Single  exp_bits=8  fraction_bits=24  quantization=Truncate  overflow=Wrap  en=off  latency=1  dbl_ovrd=off  pipeline=on  block_type=convert
  convert1 : xbsIndex_r4/Convert  gui_display_data_type=Fixed-point  arith_type="Signed  (2's comp)"  n_bits=37  bin_pt=34  float_type=Single  exp_bits=8  fraction_bits=24  quantization=Truncate  overflow=Wrap  en=off  latency=1  dbl_ovrd=off  pipeline=on  block_type=convert
  mults : Subsystem
  c : Outport
  wires:
  a_input_c_to_ri/1(re) -> mults/7(a4), mults/1(a1)  "a_re"
  b_input_c_to_ri/1(re) -> mults/6(b3), mults/2(b1)  "b_re"
  a_input_c_to_ri/2(im) -> mults/5(a3), mults/3(a2)  "a_im"
  b_input_c_to_ri/2(im) -> mults/8(b4), mults/4(b2)  "b_im"
  convert1/1 -> c_output_ri_to_c/2(im)  "c_im"
  AddSub1/1 -> convert1/1
  convert0/1 -> c_output_ri_to_c/1(re)  "c_re"
  AddSub/1 -> convert0/1
  mults/4(c4) -> AddSub1/2
  mults/3(c3) -> AddSub1/1
  mults/2(c2) -> AddSub/2
  mults/1(c1) -> AddSub/1
  c_output_ri_to_c/1(c) -> c/1
  b/1 -> b_input_c_to_ri/1(c)
  a/1 -> a_input_c_to_ri/1(c)

== system kurtosis/kurtosis/kurtosis_origin_moments_4/ri_to_c_x_3rd ==
  re : Inport
  im : Inport  Port=2
  concat : xbsIndex_r4/Concat  num_inputs=2  dbl_ovrd=off  block_type=concat
  force_im : xbsIndex_r4/Reinterpret  force_arith_type=on  arith_type=Unsigned  force_bin_pt=on  bin_pt=0  block_type=reinterpret
  force_re : xbsIndex_r4/Reinterpret  force_arith_type=on  arith_type=Unsigned  force_bin_pt=on  bin_pt=0  block_type=reinterpret
  c : Outport
  wires:
  force_re/1 -> concat/1
  re/1 -> force_re/1
  force_im/1 -> concat/2
  im/1 -> force_im/1
  concat/1 -> c/1

== system kurtosis/kurtosis/kurtosis_origin_moments_5/abs_x_sq ==
  c : Inport
  c_to_ri : Subsystem
  imag_square : xbsIndex_r4/Mult  precision=Full  arith_type="Signed  (2's comp)"  n_bits=16  bin_pt=14  quantization=Truncate  overflow=Wrap  en=off  latency=3  dbl_ovrd=off  use_behavioral_HDL=off  opt=Speed  use_embedded=on  optimum_pipeline=off  pipeline=on  use_rpm=on  placement_style=Rectangular shape  block_type=mult
  power_adder : xbsIndex_r4/AddSub  mode=Addition  use_carryin=off  use_carryout=off  en=off  latency=2  precision=Full  arith_type=Unsigned  n_bits=16  bin_pt=14  quantization=Truncate  overflow=Wrap  dbl_ovrd=off  use_behavioral_HDL=on  hw_selection=Fabric  pipelined=off  use_rpm=on  block_type=addsub
  real_square : xbsIndex_r4/Mult  precision=Full  arith_type="Signed  (2's comp)"  n_bits=16  bin_pt=14  quantization=Truncate  overflow=Wrap  en=off  latency=3  dbl_ovrd=off  use_behavioral_HDL=off  opt=Speed  use_embedded=on  optimum_pipeline=off  pipeline=on  use_rpm=on  placement_style=Triangular  block_type=mult
  power : Outport
  wires:
  c_to_ri/2(im) -> imag_square/2, imag_square/1
  c_to_ri/1(re) -> real_square/2, real_square/1
  real_square/1 -> power_adder/1
  power_adder/1 -> power/1
  imag_square/1 -> power_adder/2
  c/1 -> c_to_ri/1(c)

== system kurtosis/kurtosis/kurtosis_origin_moments_5/c_to_ri_xin ==
  c : Inport
  force_im : xbsIndex_r4/Reinterpret  force_arith_type=on  arith_type="Signed  (2's comp)"  force_bin_pt=on  bin_pt=17  block_type=reinterpret
  force_re : xbsIndex_r4/Reinterpret  force_arith_type=on  arith_type="Signed  (2's comp)"  force_bin_pt=on  bin_pt=17  block_type=reinterpret
  slice_im : xbsIndex_r4/Slice  nbits=18  boolean_output=off  mode=Lower Bit Location + Width  bit1=0  base1=MSB of Input  bit0=0  base0=LSB of Input  dbl_ovrd=off  block_type=slice
  slice_re : xbsIndex_r4/Slice  nbits=18  boolean_output=off  mode=Upper Bit Location + Width  bit1=0  base1=MSB of Input  bit0=0  base0=LSB of Input  dbl_ovrd=off  block_type=slice
  re : Outport
  im : Outport  Port=2
  wires:
  c/1 -> slice_im/1, slice_re/1
  force_im/1 -> im/1
  slice_im/1 -> force_im/1
  force_re/1 -> re/1
  slice_re/1 -> force_re/1

== system kurtosis/kurtosis/kurtosis_origin_moments_5/cplx_sq ==
  a : Inport
  b : Inport  Port=2
  AddSub : xbsIndex_r4/AddSub  mode=Subtraction  use_carryin=off  use_carryout=off  en=off  latency=2  precision=Full  arith_type=Unsigned  n_bits=16  bin_pt=14  quantization=Truncate  overflow=Wrap  dbl_ovrd=off  use_behavioral_HDL=on  hw_selection=Fabric  pipelined=off  block_type=addsub
  AddSub1 : xbsIndex_r4/AddSub  mode=Addition  use_carryin=off  use_carryout=off  en=off  latency=2  precision=Full  arith_type=Unsigned  n_bits=16  bin_pt=14  quantization=Truncate  overflow=Wrap  dbl_ovrd=off  use_behavioral_HDL=on  hw_selection=Fabric  pipelined=off  block_type=addsub
  a_input_c_to_ri : Subsystem
  b_input_c_to_ri : Subsystem
  c_output_ri_to_c : Subsystem
  convert0 : xbsIndex_r4/Convert  gui_display_data_type=Fixed-point  arith_type="Signed  (2's comp)"  n_bits=37  bin_pt=34  float_type=Single  exp_bits=8  fraction_bits=24  quantization=Truncate  overflow=Wrap  en=off  latency=1  dbl_ovrd=off  pipeline=on  block_type=convert
  convert1 : xbsIndex_r4/Convert  gui_display_data_type=Fixed-point  arith_type="Signed  (2's comp)"  n_bits=37  bin_pt=34  float_type=Single  exp_bits=8  fraction_bits=24  quantization=Truncate  overflow=Wrap  en=off  latency=1  dbl_ovrd=off  pipeline=on  block_type=convert
  mults : Subsystem
  c : Outport
  wires:
  a_input_c_to_ri/1(re) -> mults/7(a4), mults/1(a1)  "a_re"
  b_input_c_to_ri/1(re) -> mults/6(b3), mults/2(b1)  "b_re"
  a_input_c_to_ri/2(im) -> mults/5(a3), mults/3(a2)  "a_im"
  b_input_c_to_ri/2(im) -> mults/8(b4), mults/4(b2)  "b_im"
  convert1/1 -> c_output_ri_to_c/2(im)  "c_im"
  AddSub1/1 -> convert1/1
  convert0/1 -> c_output_ri_to_c/1(re)  "c_re"
  AddSub/1 -> convert0/1
  mults/4(c4) -> AddSub1/2
  mults/3(c3) -> AddSub1/1
  mults/2(c2) -> AddSub/2
  mults/1(c1) -> AddSub/1
  c_output_ri_to_c/1(c) -> c/1
  b/1 -> b_input_c_to_ri/1(c)
  a/1 -> a_input_c_to_ri/1(c)

== system kurtosis/kurtosis/kurtosis_origin_moments_5/ri_to_c_x_3rd ==
  re : Inport
  im : Inport  Port=2
  concat : xbsIndex_r4/Concat  num_inputs=2  dbl_ovrd=off  block_type=concat
  force_im : xbsIndex_r4/Reinterpret  force_arith_type=on  arith_type=Unsigned  force_bin_pt=on  bin_pt=0  block_type=reinterpret
  force_re : xbsIndex_r4/Reinterpret  force_arith_type=on  arith_type=Unsigned  force_bin_pt=on  bin_pt=0  block_type=reinterpret
  c : Outport
  wires:
  force_re/1 -> concat/1
  re/1 -> force_re/1
  force_im/1 -> concat/2
  im/1 -> force_im/1
  concat/1 -> c/1

== system kurtosis/kurtosis/kurtosis_origin_moments_6/abs_x_sq ==
  c : Inport
  c_to_ri : Subsystem
  imag_square : xbsIndex_r4/Mult  precision=Full  arith_type="Signed  (2's comp)"  n_bits=16  bin_pt=14  quantization=Truncate  overflow=Wrap  en=off  latency=3  dbl_ovrd=off  use_behavioral_HDL=off  opt=Speed  use_embedded=on  optimum_pipeline=off  pipeline=on  use_rpm=on  placement_style=Rectangular shape  block_type=mult
  power_adder : xbsIndex_r4/AddSub  mode=Addition  use_carryin=off  use_carryout=off  en=off  latency=2  precision=Full  arith_type=Unsigned  n_bits=16  bin_pt=14  quantization=Truncate  overflow=Wrap  dbl_ovrd=off  use_behavioral_HDL=on  hw_selection=Fabric  pipelined=off  use_rpm=on  block_type=addsub
  real_square : xbsIndex_r4/Mult  precision=Full  arith_type="Signed  (2's comp)"  n_bits=16  bin_pt=14  quantization=Truncate  overflow=Wrap  en=off  latency=3  dbl_ovrd=off  use_behavioral_HDL=off  opt=Speed  use_embedded=on  optimum_pipeline=off  pipeline=on  use_rpm=on  placement_style=Triangular  block_type=mult
  power : Outport
  wires:
  c_to_ri/2(im) -> imag_square/2, imag_square/1
  c_to_ri/1(re) -> real_square/2, real_square/1
  real_square/1 -> power_adder/1
  power_adder/1 -> power/1
  imag_square/1 -> power_adder/2
  c/1 -> c_to_ri/1(c)

== system kurtosis/kurtosis/kurtosis_origin_moments_6/c_to_ri_xin ==
  c : Inport
  force_im : xbsIndex_r4/Reinterpret  force_arith_type=on  arith_type="Signed  (2's comp)"  force_bin_pt=on  bin_pt=17  block_type=reinterpret
  force_re : xbsIndex_r4/Reinterpret  force_arith_type=on  arith_type="Signed  (2's comp)"  force_bin_pt=on  bin_pt=17  block_type=reinterpret
  slice_im : xbsIndex_r4/Slice  nbits=18  boolean_output=off  mode=Lower Bit Location + Width  bit1=0  base1=MSB of Input  bit0=0  base0=LSB of Input  dbl_ovrd=off  block_type=slice
  slice_re : xbsIndex_r4/Slice  nbits=18  boolean_output=off  mode=Upper Bit Location + Width  bit1=0  base1=MSB of Input  bit0=0  base0=LSB of Input  dbl_ovrd=off  block_type=slice
  re : Outport
  im : Outport  Port=2
  wires:
  c/1 -> slice_im/1, slice_re/1
  force_im/1 -> im/1
  slice_im/1 -> force_im/1
  force_re/1 -> re/1
  slice_re/1 -> force_re/1

== system kurtosis/kurtosis/kurtosis_origin_moments_6/cplx_sq ==
  a : Inport
  b : Inport  Port=2
  AddSub : xbsIndex_r4/AddSub  mode=Subtraction  use_carryin=off  use_carryout=off  en=off  latency=2  precision=Full  arith_type=Unsigned  n_bits=16  bin_pt=14  quantization=Truncate  overflow=Wrap  dbl_ovrd=off  use_behavioral_HDL=on  hw_selection=Fabric  pipelined=off  block_type=addsub
  AddSub1 : xbsIndex_r4/AddSub  mode=Addition  use_carryin=off  use_carryout=off  en=off  latency=2  precision=Full  arith_type=Unsigned  n_bits=16  bin_pt=14  quantization=Truncate  overflow=Wrap  dbl_ovrd=off  use_behavioral_HDL=on  hw_selection=Fabric  pipelined=off  block_type=addsub
  a_input_c_to_ri : Subsystem
  b_input_c_to_ri : Subsystem
  c_output_ri_to_c : Subsystem
  convert0 : xbsIndex_r4/Convert  gui_display_data_type=Fixed-point  arith_type="Signed  (2's comp)"  n_bits=37  bin_pt=34  float_type=Single  exp_bits=8  fraction_bits=24  quantization=Truncate  overflow=Wrap  en=off  latency=1  dbl_ovrd=off  pipeline=on  block_type=convert
  convert1 : xbsIndex_r4/Convert  gui_display_data_type=Fixed-point  arith_type="Signed  (2's comp)"  n_bits=37  bin_pt=34  float_type=Single  exp_bits=8  fraction_bits=24  quantization=Truncate  overflow=Wrap  en=off  latency=1  dbl_ovrd=off  pipeline=on  block_type=convert
  mults : Subsystem
  c : Outport
  wires:
  a_input_c_to_ri/1(re) -> mults/7(a4), mults/1(a1)  "a_re"
  b_input_c_to_ri/1(re) -> mults/6(b3), mults/2(b1)  "b_re"
  a_input_c_to_ri/2(im) -> mults/5(a3), mults/3(a2)  "a_im"
  b_input_c_to_ri/2(im) -> mults/8(b4), mults/4(b2)  "b_im"
  convert1/1 -> c_output_ri_to_c/2(im)  "c_im"
  AddSub1/1 -> convert1/1
  convert0/1 -> c_output_ri_to_c/1(re)  "c_re"
  AddSub/1 -> convert0/1
  mults/4(c4) -> AddSub1/2
  mults/3(c3) -> AddSub1/1
  mults/2(c2) -> AddSub/2
  mults/1(c1) -> AddSub/1
  c_output_ri_to_c/1(c) -> c/1
  b/1 -> b_input_c_to_ri/1(c)
  a/1 -> a_input_c_to_ri/1(c)

== system kurtosis/kurtosis/kurtosis_origin_moments_6/ri_to_c_x_3rd ==
  re : Inport
  im : Inport  Port=2
  concat : xbsIndex_r4/Concat  num_inputs=2  dbl_ovrd=off  block_type=concat
  force_im : xbsIndex_r4/Reinterpret  force_arith_type=on  arith_type=Unsigned  force_bin_pt=on  bin_pt=0  block_type=reinterpret
  force_re : xbsIndex_r4/Reinterpret  force_arith_type=on  arith_type=Unsigned  force_bin_pt=on  bin_pt=0  block_type=reinterpret
  c : Outport
  wires:
  force_re/1 -> concat/1
  re/1 -> force_re/1
  force_im/1 -> concat/2
  im/1 -> force_im/1
  concat/1 -> c/1

== system kurtosis/kurtosis/kurtosis_origin_moments_7/abs_x_sq ==
  c : Inport
  c_to_ri : Subsystem
  imag_square : xbsIndex_r4/Mult  precision=Full  arith_type="Signed  (2's comp)"  n_bits=16  bin_pt=14  quantization=Truncate  overflow=Wrap  en=off  latency=3  dbl_ovrd=off  use_behavioral_HDL=off  opt=Speed  use_embedded=on  optimum_pipeline=off  pipeline=on  use_rpm=on  placement_style=Rectangular shape  block_type=mult
  power_adder : xbsIndex_r4/AddSub  mode=Addition  use_carryin=off  use_carryout=off  en=off  latency=2  precision=Full  arith_type=Unsigned  n_bits=16  bin_pt=14  quantization=Truncate  overflow=Wrap  dbl_ovrd=off  use_behavioral_HDL=on  hw_selection=Fabric  pipelined=off  use_rpm=on  block_type=addsub
  real_square : xbsIndex_r4/Mult  precision=Full  arith_type="Signed  (2's comp)"  n_bits=16  bin_pt=14  quantization=Truncate  overflow=Wrap  en=off  latency=3  dbl_ovrd=off  use_behavioral_HDL=off  opt=Speed  use_embedded=on  optimum_pipeline=off  pipeline=on  use_rpm=on  placement_style=Triangular  block_type=mult
  power : Outport
  wires:
  c_to_ri/2(im) -> imag_square/2, imag_square/1
  c_to_ri/1(re) -> real_square/2, real_square/1
  real_square/1 -> power_adder/1
  power_adder/1 -> power/1
  imag_square/1 -> power_adder/2
  c/1 -> c_to_ri/1(c)

== system kurtosis/kurtosis/kurtosis_origin_moments_7/c_to_ri_xin ==
  c : Inport
  force_im : xbsIndex_r4/Reinterpret  force_arith_type=on  arith_type="Signed  (2's comp)"  force_bin_pt=on  bin_pt=17  block_type=reinterpret
  force_re : xbsIndex_r4/Reinterpret  force_arith_type=on  arith_type="Signed  (2's comp)"  force_bin_pt=on  bin_pt=17  block_type=reinterpret
  slice_im : xbsIndex_r4/Slice  nbits=18  boolean_output=off  mode=Lower Bit Location + Width  bit1=0  base1=MSB of Input  bit0=0  base0=LSB of Input  dbl_ovrd=off  block_type=slice
  slice_re : xbsIndex_r4/Slice  nbits=18  boolean_output=off  mode=Upper Bit Location + Width  bit1=0  base1=MSB of Input  bit0=0  base0=LSB of Input  dbl_ovrd=off  block_type=slice
  re : Outport
  im : Outport  Port=2
  wires:
  c/1 -> slice_im/1, slice_re/1
  force_im/1 -> im/1
  slice_im/1 -> force_im/1
  force_re/1 -> re/1
  slice_re/1 -> force_re/1
